simulink model "indicator_logic"  (R2024b)
settings: Solver=FixedStepDiscrete  StartTime=0.0  StopTime=inf  FixedStep=0.1  RelTol=1e-3
settings Model: Creator=ashba  LastModifiedBy=Shaik Abdul Khadir
settings OptimizationCC: DefaultParameterBehavior=Inlined  EnhancedBackFolding=on  PassReuseOutputArgsAs=Individual arguments  ZeroExternalMemoryAtStartup=off  ZeroInternalMemoryAtStartup=off  OptimizeBlockOrder=speed  DifferentSizesBufferReuse=on  OptimizationCustomize=off  EfficientTunableParamExpr=on
settings DebuggingCC: ParameterTunabilityLossMsg=error
settings SFSimCC: MATLABDynamicMemAlloc=off
settings RTWCC: Description=Embedded Coder  SystemTargetFile=ert.tlc  GenCodeOnly=on  TemplateMakefile=ert_default_tmf  DataTypeReplacement=CDataTypesFixedWidth
settings CodeAppCC: ForceParamTrailComments=on  IgnoreCustomStorageClasses=off  OperatorAnnotations=on  SimulinkDataObjDesc=on  SFDataObjDesc=on  InsertBlockDesc=on
settings ERTTargetCC: TargetLangStandard=C99 (ISO)  GenerateSampleERTMain=on  ERTCustomFileTemplate=example_file_process.tlc  MaxIdInt64=INT64_MAX  MinIdInt64=INT64_MIN  MaxIdUint64=UINT64_MAX  MaxIdInt32=INT32_MAX  MinIdInt32=INT32_MIN  MaxIdUint32=UINT32_MAX  MaxIdInt16=INT16_MAX  MinIdInt16=INT16_MIN  MaxIdUint16=UINT16_MAX  MaxIdInt8=INT8_MAX  MinIdInt8=INT8_MIN  MaxIdUint8=UINT8_MAX

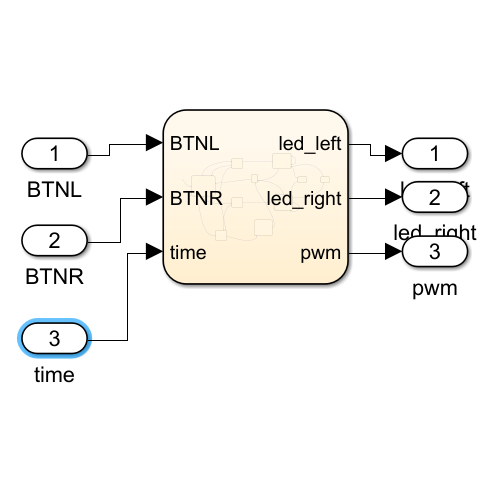
[thumbnail: Simulink's stored preview of the top-level diagram]
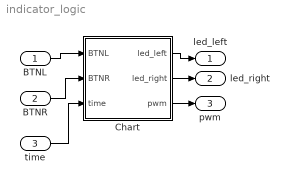
== system indicator_logic ==
  BTNL : Inport  OutDataTypeStr=uint8
  BTNR : Inport  Port=2  OutDataTypeStr=uint8
  time : Inport  Port=3  OutDataTypeStr=uint32
  Chart : Stateflow chart  TreatAsAtomicUnit=on
  led_left : Outport  OutDataTypeStr=uint8
  led_right : Outport  Port=2  OutDataTypeStr=uint8
  pwm : Outport  Port=3  OutDataTypeStr=uint8
  wires:
  Chart/1(led_left) -> led_left/1
  Chart/2(led_right) -> led_right/1
  BTNL/1 -> Chart/1(BTNL)
  BTNR/1 -> Chart/2(BTNR)
  Chart/3(pwm) -> pwm/1
  time/1 -> Chart/3(time)

== stateflow chart indicator_logic/Chart ==
  state Right
    led_left = 0;
    led_right=1;
    pwm=1;
  state Hold_1
    entry:
    entry_time = time;
  state Hold_3
    entry:
    entry_time = time;
  state Idle
    led_left = 0;
    led_right = 0;
    pwm = 0;
  state Hold_5
    entry:
    entry_time = time;
  state Hold_6
    entry:
    entry_time = time;
  state Hold_7
    entry:
    entry_time = time;
  state Hold_8
    entry:
    entry_time = time;
  state Left
    led_left = 1;
    led_right=0;
    pwm=1;
  state Hold_2
    entry:
    entry_time = time;
  state Hold_4
    entry:
    entry_time = time;
  state Hazard
    led_left = 1;
    led_right=1;
    pwm=1;
  Right -> Right [order 1] : [BTNL == 0 && BTNR == 0]
  Idle -> Hold_1 [order 1] : [BTNL == 0 && BTNR==1]
  Hold_1 -> Right [order 1] : [BTNL==0 && BTNR==0 && (time - entry_time) >= 1000]
  Hold_6 -> Right [order 1] : [BTNL==0 && BTNR==0 && (time - entry_time) >= 1000]
  Hold_1 -> Idle [order 3] : [BTNL==0 && BTNR==0 && (time - entry_time) < 1000]
  Right -> Hold_5 [order 3] : [BTNL == 1 && BTNR == 0]
  Hold_1 -> Hold_4 [order 2] : [BTNL == 1 && BTNR==1]
  Right -> Hold_3 [order 2] : [BTNL == 0 && BTNR == 1]
  Hold_3 -> Right [order 2] : [BTNL == 0 && BTNR == 0 && (time - entry_time) < 1000]
  Hold_5 -> Right [order 2] : [BTNL == 0 && BTNR == 0 && (time - entry_time) < 1000]
  (default) -> Idle
  Hold_3 -> Idle [order 1] : [BTNL == 0 && BTNR == 0 && (time - entry_time) >= 1000]
  Hold_5 -> Left [order 1] : [BTNL==0 && BTNR==0 && (time - entry_time) >= 1000]
  Hold_6 -> Left [order 2] : [BTNL == 0 && BTNR == 0 && (time - entry_time) < 1000]
  Left -> Hold_6 [order 3] : [BTNL == 0 && BTNR == 1]
  Left -> Hold_7 [order 2] : [BTNL == 1 && BTNR == 0]
  Hold_7 -> Idle [order 1] : [BTNL==0 && BTNR==0 && (time - entry_time) >= 1000]
  Hold_7 -> Left [order 2] : [BTNL==0 && BTNR==0 && (time - entry_time) < 1000]
  Hold_8 -> Idle [order 1] : [BTNL==0 && BTNR==0 && (time - entry_time) >= 1000]
  Hold_2 -> Idle [order 2] : [BTNL==0 && BTNR==0 && (time - entry_time) < 1000]
  Idle -> Hold_4 [order 3] : [BTNL == 1 && BTNR == 1]
  Idle -> Hold_2 [order 2] : [BTNL == 1 && BTNR == 0]
  Hold_4 -> Idle [order 2] : [BTNL==0 && BTNR==0 && (time - entry_time) < 1000]
  Hold_8 -> Hazard [order 2] : [BTNL==0 && BTNR==0 && (time - entry_time) < 1000]
  Hazard -> Hold_8 : [BTNL == 1 || BTNR == 1]
  Left -> Left [order 1] : [BTNL==0 && BTNR == 0]
  Hold_2 -> Left [order 3] : [BTNL==0 && BTNR==0 && (time - entry_time) >= 1000]
  Hold_2 -> Hold_4 [order 1] : [BTNL == 1 && BTNR == 1]
  Hold_4 -> Hazard [order 1] : [BTNL == 0 && BTNR == 0 && (time - entry_time) >= 1000]
  data: led_left output uint8; led_right output uint8; BTNL input uint8; BTNR input uint8; pwm output uint8; data local; Left local; left_timer local uint8 =0; right_timer local uint8 =0; threshold_ticks constant uint8 =10; time input uint32; entry_time local
